simulink model "Optimized_wind_farm_with_dynamic_grid"  (R2015b)
settings: Solver=FixedStepAuto  StartTime=0.0  StopTime=24  FixedStep=Ts  RelTol=1e-3
undefined symbols (not defined in the file): Ts
libraries: powerlib x52, simulink x38, powerlib_meascontrol x30, powerlib_extras x4, sps_avr x1
(part 1 of 3)
settings Model: SimulationMode=accelerator  Creator=Eren  LastModifiedBy=Eren

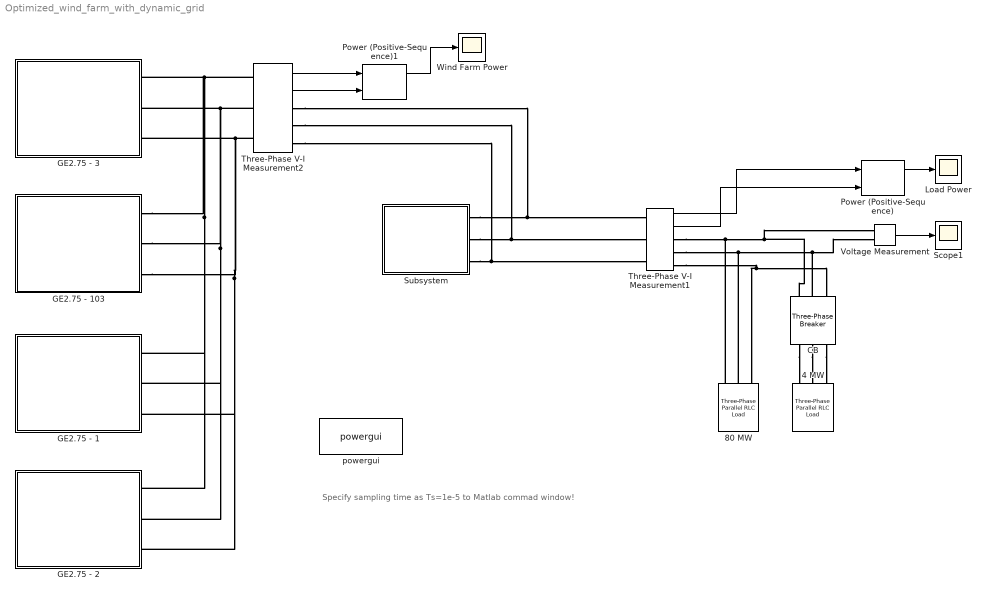
== system Optimized_wind_farm_with_dynamic_grid ==
  note: Specify sampling time as Ts=1e-5 to Matlab commad window!
  4 MW : powerlib/Elements/Three-Phase Parallel RLC Load  LConnTagsString=A|B|C  Configuration=Y (grounded)  NominalVoltage=690  Vabc=[1e3 1e3 1e3]  Vabcp=[1e3 1e3 1e3]  NominalFrequency=50  UnbalancedPower=off  ActivePower=8e6  InductivePower=0  CapacitivePower=0  Pabc=[10e3 9e3 11e3]  QLabc=[100 90 110]  QCabc=[100 90 110]  Pabcp=[10e3 9e3 11e3]  QLabcp=[100 90 110]  QCabcp=[100 90 110]  Measurements=None  LoadType=constant PQ
  80 MW : powerlib/Elements/Three-Phase Parallel RLC Load  LConnTagsString=A|B|C  Configuration=Y (grounded)  NominalVoltage=690  Vabc=[1e3 1e3 1e3]  Vabcp=[1e3 1e3 1e3]  NominalFrequency=50  UnbalancedPower=off  ActivePower=80e6  InductivePower=0  CapacitivePower=0  Pabc=[10e3 9e3 11e3]  QLabc=[100 90 110]  QCabc=[100 90 110]  Pabcp=[10e3 9e3 11e3]  QLabcp=[100 90 110]  QCabcp=[100 90 110]  Measurements=None  LoadType=constant PQ
  CB : powerlib/Elements/Three-Phase Breaker  InitialState=open  SwitchA=on  SwitchB=on  SwitchC=on  SwitchTimes=10  External=off  BreakerResistance=0.01  SnubberResistance=1e6  SnubberCapacitance=inf  Measurements=None
  GE2.75 - 1 : Subsystem  mask{Prated=2.75e6, R=51.5, windspeed=9, Jtotal=1058.2, p=1.225, startuptime=5, winit=-160, gear=117.4, wmax=2*pi*(1735/60), fluxlinkage=4, pgen=2, Ld=10e-4, Lq=10.5e-4, Rs=1e-10, drivefreq=10e3, fnom=50, Srated=3.04e6, Vdcset=2500, Cdc=27e-3, Lfilter=2e-4}
      mask prompts: Prated "Turbine Power (W)"; R "Blade Radius"; windspeed "Wind Speed"; Jtotal "Total Inertia"; p "Air Density"; startuptime "Turbine Start-up Time"; winit "Initial Generator Speed"; gear "Gearbox Ratio"; wmax "Max Generator Speed"; fluxlinkage "Flux Linkage"; pgen "Generator Pole Pairs"; Ld "Ld (H)"; Lq "Lq(H)"; Rs "Stator Resistance"; drivefreq "Drive Frequency"; fnom "Nominal Grid Frequency"; Srated "Drive Apparent Power"; Vdcset "DC Link Voltage"; Cdc "DC Link Capacitance"; Lfilter "Lfilter (H)"
      mask Display: image(imread('gepic.jpg'))
  GE2.75 - 103 : Subsystem  mask{Prated=2.75e6, R=51.5, windspeed=9, Jtotal=1058.2, p=1.225, startuptime=5, winit=-160, gear=117.4, wmax=2*pi*(1735/60), fluxlinkage=4, pgen=2, Ld=10e-4, Lq=10.5e-4, Rs=1e-10, drivefreq=10e3, fnom=50, Srated=3.04e6, Vdcset=2500, Cdc=27e-3, Lfilter=2e-4}
      mask prompts: Prated "Turbine Power (W)"; R "Blade Radius"; windspeed "Wind Speed"; Jtotal "Total Inertia"; p "Air Density"; startuptime "Turbine Start-up Time"; winit "Initial Generator Speed"; gear "Gearbox Ratio"; wmax "Max Generator Speed"; fluxlinkage "Flux Linkage"; pgen "Generator Pole Pairs"; Ld "Ld (H)"; Lq "Lq(H)"; Rs "Stator Resistance"; drivefreq "Drive Frequency"; fnom "Nominal Grid Frequency"; Srated "Drive Apparent Power"; Vdcset "DC Link Voltage"; Cdc "DC Link Capacitance"; Lfilter "Lfilter (H)"
      mask Display: image(imread('gepic.jpg'))
  GE2.75 - 2 : Subsystem  mask{Prated=2.75e6, R=51.5, windspeed=9, Jtotal=1058.2, p=1.225, startuptime=5, winit=-160, gear=117.4, wmax=2*pi*(1735/60), fluxlinkage=4, pgen=2, Ld=10e-4, Lq=10.5e-4, Rs=1e-10, drivefreq=10e3, fnom=50, Srated=3.04e6, Vdcset=2500, Cdc=27e-3, Lfilter=2e-4}
      mask prompts: Prated "Turbine Power (W)"; R "Blade Radius"; windspeed "Wind Speed"; Jtotal "Total Inertia"; p "Air Density"; startuptime "Turbine Start-up Time"; winit "Initial Generator Speed"; gear "Gearbox Ratio"; wmax "Max Generator Speed"; fluxlinkage "Flux Linkage"; pgen "Generator Pole Pairs"; Ld "Ld (H)"; Lq "Lq(H)"; Rs "Stator Resistance"; drivefreq "Drive Frequency"; fnom "Nominal Grid Frequency"; Srated "Drive Apparent Power"; Vdcset "DC Link Voltage"; Cdc "DC Link Capacitance"; Lfilter "Lfilter (H)"
      mask Display: image(imread('gepic.jpg'))
  GE2.75 - 3 : Subsystem  mask{Prated=2.75e6, R=51.5, windspeed=9, Jtotal=1058.2, p=1.225, startuptime=5, winit=-160, gear=117.4, wmax=2*pi*(1735/60), fluxlinkage=4, pgen=2, Ld=10e-4, Lq=10.5e-4, Rs=1e-10, drivefreq=10e3, fnom=50, Srated=3.04e6, Vdcset=2500, Cdc=27e-3, Lfilter=2e-4}
      mask prompts: Prated "Turbine Power (W)"; R "Blade Radius"; windspeed "Wind Speed"; Jtotal "Total Inertia"; p "Air Density"; startuptime "Turbine Start-up Time"; winit "Initial Generator Speed"; gear "Gearbox Ratio"; wmax "Max Generator Speed"; fluxlinkage "Flux Linkage"; pgen "Generator Pole Pairs"; Ld "Ld (H)"; Lq "Lq(H)"; Rs "Stator Resistance"; drivefreq "Drive Frequency"; fnom "Nominal Grid Frequency"; Srated "Drive Apparent Power"; Vdcset "DC Link Voltage"; Cdc "DC Link Capacitance"; Lfilter "Lfilter (H)"
      mask Display: image(imread('gepic.jpg'))
  Load Power : Scope
  Power (Positive-Sequence) : powerlib_meascontrol/Measurements/Power (Positive-Sequence)  Freq=50  Vinit=[0, 0]  Iinit=[0, 0]  Ts=0
  Power (Positive-Sequence)1 : powerlib_meascontrol/Measurements/Power (Positive-Sequence)  Freq=50  Vinit=[0, 0]  Iinit=[0, 0]  Ts=0
  Scope1 : Scope
  Subsystem : Subsystem
  Three-Phase V-I Measurement1 : powerlib/Measurements/Three-Phase V-I Measurement  VoltageMeasurement=phase-to-ground  SetLabelV=off  LabelV=Vsabc  Vpu=off  VpuLL=on  CurrentMeasurement=yes  SetLabelI=off  LabelI=Isabc  Ipu=off  Pbase=100e6  Vbase=690  OutputType=Complex  PhasorSimulation=off  PSBequivalent=0
  Three-Phase V-I Measurement2 : powerlib/Measurements/Three-Phase V-I Measurement  VoltageMeasurement=phase-to-ground  SetLabelV=off  LabelV=Vsabc  Vpu=off  VpuLL=on  CurrentMeasurement=yes  SetLabelI=off  LabelI=Isabc  Ipu=off  Pbase=100e6  Vbase=690  OutputType=Complex  PhasorSimulation=off  PSBequivalent=0
  Voltage Measurement : powerlib/Measurements/Voltage Measurement  PhasorSimulation=off  OutputType=Complex  PSBequivalent=0
  Wind Farm Power : Scope
  powergui : powerlib/powergui  Priority=2  SimulationMode=Discrete  SolverType=Tustin  SampleTime=Ts  frequency=60  SPID=off  DisableSnubberDevices=off  DisableRonSwitches=off  DisableVfSwitches=off  SwTol=0  DisplayEquations=off  Interpol=off  ExternalGateDelay=off  methode=off  Ts=0  FunctionMessages=off  echomessages=off  HookPort=off  EnableUseOfTLC=off  x0status=blocks  frequencyindice=50  Pbase=100e6  ErrMax=1e-4  Iterations=50  UnitsV=kV  UnitsW=MW  buscounter=0  RestoreLinks=warning  ResistiveCurrentMeasurement=off  Frange=[0:2:500]  Ylog=off  Xlog=on  ShowGrid=off  save=off  variable=ZData  structure=0  ZoomFFT=on  StartTime=0.0  cycles=1  DisplayStyle=1  fundamental=60  FreqAxis=off  MaxFrequency=1000  frequencyindicesteady=1  RmsSteady=1  display=off
  wires:
  Voltage Measurement/1 -> Scope1/1
  Three-Phase V-I Measurement1/1 -> Power (Positive-Sequence)/1
  Three-Phase V-I Measurement1/2 -> Power (Positive-Sequence)/2
  Power (Positive-Sequence)/1 -> Load Power/1
  Power (Positive-Sequence)1/1 -> Wind Farm Power/1
  Three-Phase V-I Measurement2/1 -> Power (Positive-Sequence)1/1
  Three-Phase V-I Measurement2/2 -> Power (Positive-Sequence)1/2
  connections:
  80 MW/LConn1 -- CB/RConn1 -- Voltage Measurement/LConn1 -- Three-Phase V-I Measurement1/RConn1
  80 MW/LConn2 -- CB/RConn2 -- Voltage Measurement/LConn2 -- Three-Phase V-I Measurement1/RConn2
  Three-Phase V-I Measurement1/RConn3 -- CB/RConn3 -- 80 MW/LConn3
  CB/LConn2 -- 4 MW/LConn2
  CB/LConn1 -- 4 MW/LConn1
  CB/LConn3 -- 4 MW/LConn3
  Subsystem/RConn3 -- Three-Phase V-I Measurement2/RConn3 -- Three-Phase V-I Measurement1/LConn3
  Subsystem/RConn1 -- Three-Phase V-I Measurement2/RConn1 -- Three-Phase V-I Measurement1/LConn1
  Subsystem/RConn2 -- Three-Phase V-I Measurement1/LConn2 -- Three-Phase V-I Measurement2/RConn2
  Three-Phase V-I Measurement2/LConn1 -- GE2.75 - 103/RConn1 -- GE2.75 - 2/RConn1 -- GE2.75 - 1/RConn1 -- GE2.75 - 3/RConn1
  Three-Phase V-I Measurement2/LConn2 -- GE2.75 - 103/RConn2 -- GE2.75 - 2/RConn2 -- GE2.75 - 1/RConn2 -- GE2.75 - 3/RConn2
  Three-Phase V-I Measurement2/LConn3 -- GE2.75 - 103/RConn3 -- GE2.75 - 2/RConn3 -- GE2.75 - 1/RConn3 -- GE2.75 - 3/RConn3

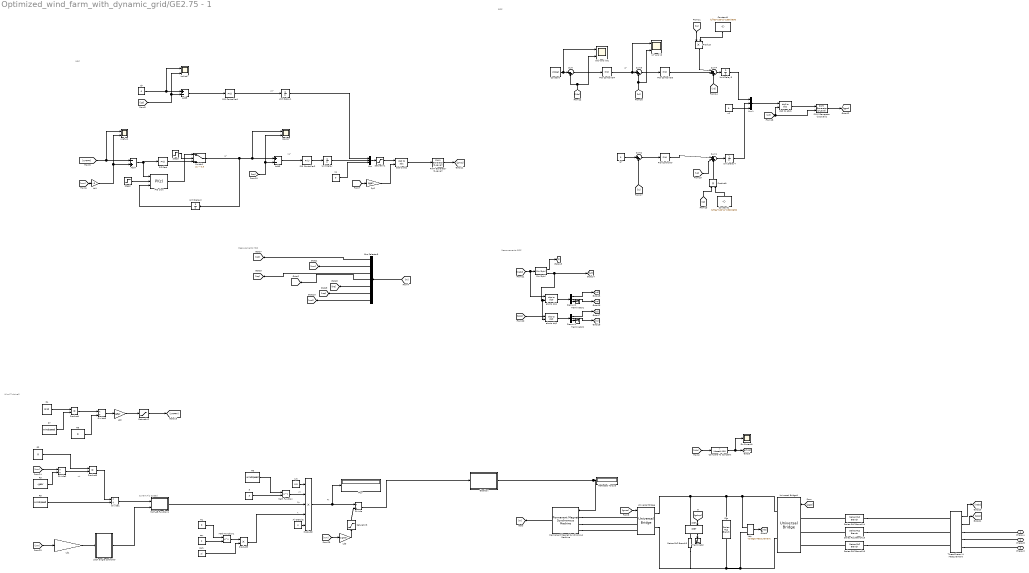
== system Optimized_wind_farm_with_dynamic_grid/GE2.75 - 1 ==
  note: Wind Turbine2
  note: Measurements GSC
  note: GSC
  note: MSC
  note: Measurements MSC
  note: Vd*
  note: Vq*
  note: iq*
  note: id*
  note: Current Tip Speed
  note: wt
  note: A
  note: Cp
  note: v3
  note: Pt
  1/2 : Constant  Value=0.5
  3 : Constant  Value=3
  Add3 : Sum  Inputs=+-
  Add5 : Sum  Inputs=+-
  Add7 : Sum  Inputs=-+
  Air Density : Constant  Value=p
  Bus Selector5 : BusSelector  OutputSignals=Stator current is_d (A),Rotor speed wm (rad/s),Stator current is_q (A),Rotor angle thetam (rad),Electromagnetic torque Te (N*m),Stator voltage Vs_q (V),Stator voltage Vs_d (V)
  Cdc : powerlib/Elements/Series RLC Branch  LConnTagsString=__new0  RConnTagsString=__new0  BranchType=C  Resistance=1  Inductance=1e-4  SetiL0=off  InitialCurrent=0  Capacitance=Cdc  Setx0=off  InitialVoltage=0  Measurements=None
  Compare To Constant : simulink/Logic and Bit Operations/Compare To Constant  relop=>  const=Vdcset+100  OutDataTypeStr=boolean
  Constant : Constant  Value=Vdcset
  Constant1 : Constant  Value=(Lfilter*100*pi*2300)/690
  Constant2 : Constant  Value=(Lfilter*100*pi*2300)/690
  Dc Current1 : Scope
  Demux1 : Demux  Outputs=3
  Demux2 : Demux  Outputs=3
  Divide{,1..3} (4 alike) : Product  Inputs=*/
  Gearbox : Subsystem
  IGBT : powerlib/Power Electronics/IGBT  Ron=0.001  Lon=0  Vf=1  Tf=1e-6  Tt=2e-6  IC=0  Rs=1e5  Cs=inf  Measurements=on
  Id* : Constant  Value=0
  Ld1 : Gain  Gain=-pgen/(2*fnom*pi)
  Ld2 : Gain  Gain=gear
  Ld3 : Gain  Gain=-1/gear
  Ld4 : Gain  Gain=-1
  MATLAB Function1 : MATLAB Function  TreatAsAtomicUnit=on
  Math Function : Math  Operator=pow  SaturateOnIntegerOverflow=on
  Math Function1 : Math  Operator=pow  SaturateOnIntegerOverflow=on
  Mux : Mux  Inputs=3
  Mux1 : Mux  Inputs=3
  PID Controller : simulink/Continuous/PID Controller  Controller=PI  TimeDomain=Continuous-time  SampleTime=-1  IntegratorMethod=Forward Euler  FilterMethod=Forward Euler  Form=Parallel  UseFilter=on  ControllerParametersSource=internal  P=15  I=1  D=0  N=100  InitialConditionSource=internal  InitialConditionForIntegrator=0  InitialConditionForFilter=0  ExternalReset=none  LimitOutput=on  UpperSaturationLimit=2  LowerSaturationLimit=-2  LinearizeAsGain=on  AntiWindupMode=none  Kb=1  TrackingMode=off  Kt=1  PParamMin=[]  PParamMax=[]  IParamMin=[]  IParamMax=[]  DParamMin=[]  DParamMax=[]  NParamMin=[]  NParamMax=[]  KbParamMin=[]  KbParamMax=[]  KtParamMin=[]  KtParamMax=[]  POutMin=[]  POutMax=[]  IOutMin=[]  IOutMax=[]  DOutMin=[]  DOutMax=[]  NOutMin=[]  NOutMax=[]  KbOutMin=[]  KbOutMax=[]  KtOutMin=[]  KtOutMax=[]  IntegratorOutMin=[]  IntegratorOutMax=[]  FilterOutMin=[]  FilterOutMax=[]  SumOutMin=[]  SumOutMax=[]  SumI1OutMin=[]  SumI1OutMax=[]  SumI2OutMin=[]  SumI2OutMax=[]  SumI3OutMin=[]  SumI3OutMax=[]  SumDOutMin=[]  SumDOutMax=[]  SaturationOutMin=[]  SaturationOutMax=[]  IntegratorContinuousStateAttributes=''  IntegratorStateMustResolveToSignalObject=off  IntegratorRTWStateStorageClass=Auto  FilterContinuousStateAttributes=''  FilterStateMustResolveToSignalObject=off  FilterRTWStateStorageClass=Auto  DifferentiatorICPrevScaledInput=0  DifferentiatorOutMin=[]  DifferentiatorOutMax=[]
  PID Controller1 : simulink/Continuous/PID Controller  Controller=PI  TimeDomain=Discrete-time  SampleTime=-1  IntegratorMethod=Forward Euler  FilterMethod=Forward Euler  Form=Parallel  UseFilter=on  ControllerParametersSource=internal  P=0.25  I=0.05  D=0  N=100  InitialConditionSource=internal  InitialConditionForIntegrator=0  InitialConditionForFilter=0  ExternalReset=none  LimitOutput=off  UpperSaturationLimit=inf  LowerSaturationLimit=-inf  LinearizeAsGain=on  AntiWindupMode=none  Kb=1  TrackingMode=off  Kt=1  PParamMin=[]  PParamMax=[]  IParamMin=[]  IParamMax=[]  DParamMin=[]  DParamMax=[]  NParamMin=[]  NParamMax=[]  KbParamMin=[]  KbParamMax=[]  KtParamMin=[]  KtParamMax=[]  POutMin=[]  POutMax=[]  IOutMin=[]  IOutMax=[]  DOutMin=[]  DOutMax=[]  NOutMin=[]  NOutMax=[]  KbOutMin=[]  KbOutMax=[]  KtOutMin=[]  KtOutMax=[]  IntegratorOutMin=[]  IntegratorOutMax=[]  FilterOutMin=[]  FilterOutMax=[]  SumOutMin=[]  SumOutMax=[]  SumI1OutMin=[]  SumI1OutMax=[]  SumI2OutMin=[]  SumI2OutMax=[]  SumI3OutMin=[]  SumI3OutMax=[]  SumDOutMin=[]  SumDOutMax=[]  SaturationOutMin=[]  SaturationOutMax=[]  IntegratorContinuousStateAttributes=''  IntegratorStateMustResolveToSignalObject=off  IntegratorRTWStateStorageClass=Auto  FilterContinuousStateAttributes=''  FilterStateMustResolveToSignalObject=off  FilterRTWStateStorageClass=Auto  DifferentiatorICPrevScaledInput=0  DifferentiatorOutMin=[]  DifferentiatorOutMax=[]
  PID Controller2 : simulink/Continuous/PID Controller  Controller=PI  TimeDomain=Discrete-time  SampleTime=-1  IntegratorMethod=Forward Euler  FilterMethod=Forward Euler  Form=Parallel  UseFilter=on  ControllerParametersSource=internal  P=1  I=0.05  D=0  N=100  InitialConditionSource=internal  InitialConditionForIntegrator=0  InitialConditionForFilter=0  ExternalReset=none  LimitOutput=off  UpperSaturationLimit=inf  LowerSaturationLimit=-inf  LinearizeAsGain=on  AntiWindupMode=none  Kb=1  TrackingMode=off  Kt=1  PParamMin=[]  PParamMax=[]  IParamMin=[]  IParamMax=[]  DParamMin=[]  DParamMax=[]  NParamMin=[]  NParamMax=[]  KbParamMin=[]  KbParamMax=[]  KtParamMin=[]  KtParamMax=[]  POutMin=[]  POutMax=[]  IOutMin=[]  IOutMax=[]  DOutMin=[]  DOutMax=[]  NOutMin=[]  NOutMax=[]  KbOutMin=[]  KbOutMax=[]  KtOutMin=[]  KtOutMax=[]  IntegratorOutMin=[]  IntegratorOutMax=[]  FilterOutMin=[]  FilterOutMax=[]  SumOutMin=[]  SumOutMax=[]  SumI1OutMin=[]  SumI1OutMax=[]  SumI2OutMin=[]  SumI2OutMax=[]  SumI3OutMin=[]  SumI3OutMax=[]  SumDOutMin=[]  SumDOutMax=[]  SaturationOutMin=[]  SaturationOutMax=[]  IntegratorContinuousStateAttributes=''  IntegratorStateMustResolveToSignalObject=off  IntegratorRTWStateStorageClass=Auto  FilterContinuousStateAttributes=''  FilterStateMustResolveToSignalObject=off  FilterRTWStateStorageClass=Auto  DifferentiatorICPrevScaledInput=0  DifferentiatorOutMin=[]  DifferentiatorOutMax=[]
  PID Controller3 : simulink/Continuous/PID Controller  Controller=PI  TimeDomain=Continuous-time  SampleTime=-1  IntegratorMethod=Forward Euler  FilterMethod=Forward Euler  Form=Parallel  UseFilter=on  ControllerParametersSource=internal  P=100  I=5  D=0  N=100  InitialConditionSource=internal  InitialConditionForIntegrator=0  InitialConditionForFilter=0  ExternalReset=none  LimitOutput=on  UpperSaturationLimit=1.5  LowerSaturationLimit=-1.5  LinearizeAsGain=on  AntiWindupMode=none  Kb=1  TrackingMode=off  Kt=1  PParamMin=[]  PParamMax=[]  IParamMin=[]  IParamMax=[]  DParamMin=[]  DParamMax=[]  NParamMin=[]  NParamMax=[]  KbParamMin=[]  KbParamMax=[]  KtParamMin=[]  KtParamMax=[]  POutMin=[]  POutMax=[]  IOutMin=[]  IOutMax=[]  DOutMin=[]  DOutMax=[]  NOutMin=[]  NOutMax=[]  KbOutMin=[]  KbOutMax=[]  KtOutMin=[]  KtOutMax=[]  IntegratorOutMin=[]  IntegratorOutMax=[]  FilterOutMin=[]  FilterOutMax=[]  SumOutMin=[]  SumOutMax=[]  SumI1OutMin=[]  SumI1OutMax=[]  SumI2OutMin=[]  SumI2OutMax=[]  SumI3OutMin=[]  SumI3OutMax=[]  SumDOutMin=[]  SumDOutMax=[]  SaturationOutMin=[]  SaturationOutMax=[]  IntegratorContinuousStateAttributes=''  IntegratorStateMustResolveToSignalObject=off  IntegratorRTWStateStorageClass=Auto  FilterContinuousStateAttributes=''  FilterStateMustResolveToSignalObject=off  FilterRTWStateStorageClass=Auto  DifferentiatorICPrevScaledInput=0  DifferentiatorOutMin=[]  DifferentiatorOutMax=[]
  PID Controller4 : simulink/Continuous/PID Controller  Controller=PI  TimeDomain=Continuous-time  SampleTime=-1  IntegratorMethod=Forward Euler  FilterMethod=Forward Euler  Form=Parallel  UseFilter=on  ControllerParametersSource=internal  P=0.004  I=0.04  D=0  N=100  InitialConditionSource=internal  InitialConditionForIntegrator=0  InitialConditionForFilter=0  ExternalReset=none  LimitOutput=on  UpperSaturationLimit=1.2  LowerSaturationLimit=1e-6  LinearizeAsGain=on  AntiWindupMode=none  Kb=1  TrackingMode=off  Kt=1  PParamMin=[]  PParamMax=[]  IParamMin=[]  IParamMax=[]  DParamMin=[]  DParamMax=[]  NParamMin=[]  NParamMax=[]  KbParamMin=[]  KbParamMax=[]  KtParamMin=[]  KtParamMax=[]  POutMin=[]  POutMax=[]  IOutMin=[]  IOutMax=[]  DOutMin=[]  DOutMax=[]  NOutMin=[]  NOutMax=[]  KbOutMin=[]  KbOutMax=[]  KtOutMin=[]  KtOutMax=[]  IntegratorOutMin=[]  IntegratorOutMax=[]  FilterOutMin=[]  FilterOutMax=[]  SumOutMin=[]  SumOutMax=[]  SumI1OutMin=[]  SumI1OutMax=[]  SumI2OutMin=[]  SumI2OutMax=[]  SumI3OutMin=[]  SumI3OutMax=[]  SumDOutMin=[]  SumDOutMax=[]  SaturationOutMin=[]  SaturationOutMax=[]  IntegratorContinuousStateAttributes=''  IntegratorStateMustResolveToSignalObject=off  IntegratorRTWStateStorageClass=Auto  FilterContinuousStateAttributes=''  FilterStateMustResolveToSignalObject=off  FilterRTWStateStorageClass=Auto  DifferentiatorICPrevScaledInput=0  DifferentiatorOutMin=[]  DifferentiatorOutMax=[]
  PID fast : simulink/Continuous/PID Controller  Controller=PI  TimeDomain=Discrete-time  SampleTime=-1  IntegratorMethod=Forward Euler  FilterMethod=Forward Euler  Form=Parallel  UseFilter=on  ControllerParametersSource=internal  P=750  I=1000  D=0  N=100  InitialConditionSource=internal  InitialConditionForIntegrator=0  InitialConditionForFilter=0  ExternalReset=none  LimitOutput=on  UpperSaturationLimit=1255  LowerSaturationLimit=200  LinearizeAsGain=on  AntiWindupMode=none  Kb=1  TrackingMode=off  Kt=1  PParamMin=[]  PParamMax=[]  IParamMin=[]  IParamMax=[]  DParamMin=[]  DParamMax=[]  NParamMin=[]  NParamMax=[]  KbParamMin=[]  KbParamMax=[]  KtParamMin=[]  KtParamMax=[]  POutMin=[]  POutMax=[]  IOutMin=[]  IOutMax=[]  DOutMin=[]  DOutMax=[]  NOutMin=[]  NOutMax=[]  KbOutMin=[]  KbOutMax=[]  KtOutMin=[]  KtOutMax=[]  IntegratorOutMin=[]  IntegratorOutMax=[]  FilterOutMin=[]  FilterOutMax=[]  SumOutMin=[]  SumOutMax=[]  SumI1OutMin=[]  SumI1OutMax=[]  SumI2OutMin=[]  SumI2OutMax=[]  SumI3OutMin=[]  SumI3OutMax=[]  SumDOutMin=[]  SumDOutMax=[]  SaturationOutMin=[]  SaturationOutMax=[]  IntegratorContinuousStateAttributes=''  IntegratorStateMustResolveToSignalObject=off  IntegratorRTWStateStorageClass=Auto  FilterContinuousStateAttributes=''  FilterStateMustResolveToSignalObject=off  FilterRTWStateStorageClass=Auto  DifferentiatorICPrevScaledInput=0  DifferentiatorOutMin=[]  DifferentiatorOutMax=[]
  PID slow : simulink/Continuous/PID Controller  Controller=PI  TimeDomain=Discrete-time  SampleTime=-1  IntegratorMethod=Forward Euler  FilterMethod=Forward Euler  Form=Parallel  UseFilter=on  ControllerParametersSource=internal  P=30  I=1.6  D=0  N=100  InitialConditionSource=external  InitialConditionForIntegrator=0  InitialConditionForFilter=0  ExternalReset=rising  LimitOutput=on  UpperSaturationLimit=1255  LowerSaturationLimit=200  LinearizeAsGain=on  AntiWindupMode=none  Kb=1  TrackingMode=off  Kt=1  PParamMin=[]  PParamMax=[]  IParamMin=[]  IParamMax=[]  DParamMin=[]  DParamMax=[]  NParamMin=[]  NParamMax=[]  KbParamMin=[]  KbParamMax=[]  KtParamMin=[]  KtParamMax=[]  POutMin=[]  POutMax=[]  IOutMin=[]  IOutMax=[]  DOutMin=[]  DOutMax=[]  NOutMin=[]  NOutMax=[]  KbOutMin=[]  KbOutMax=[]  KtOutMin=[]  KtOutMax=[]  IntegratorOutMin=[]  IntegratorOutMax=[]  FilterOutMin=[]  FilterOutMax=[]  SumOutMin=[]  SumOutMax=[]  SumI1OutMin=[]  SumI1OutMax=[]  SumI2OutMin=[]  SumI2OutMax=[]  SumI3OutMin=[]  SumI3OutMax=[]  SumDOutMin=[]  SumDOutMax=[]  SaturationOutMin=[]  SaturationOutMax=[]  IntegratorContinuousStateAttributes=''  IntegratorStateMustResolveToSignalObject=off  IntegratorRTWStateStorageClass=Auto  FilterContinuousStateAttributes=''  FilterStateMustResolveToSignalObject=off  FilterRTWStateStorageClass=Auto  DifferentiatorICPrevScaledInput=0  DifferentiatorOutMin=[]  DifferentiatorOutMax=[]
  PLL (3ph) : powerlib_meascontrol/PLL/PLL (3ph)  Fmin=45  Par_Init=[0, 50]  ParK=[180, 3200, 1]  TcD=1e-4  MaxRateChangeFreq=12  FilterCutOffFreq=25  Ts=Ts  AGC=on
  PWM Generator (2-Level) : powerlib_meascontrol/Pulse & Signal Generators/PWM Generator (2-Level)  ModulatorType=Three-phase bridge (6 pulses)  ModulatorMode=Unsynchronized  Fc=drivefreq  Pc=90  nF=60  MinMax="[ -1  1 ]"  SamplingTechnique=Natural  ModulatingSignals=off  m=0.8  Freq=60  Phase=0  Ts=Ts  ShowCarrierOutport=off
  PWM Generator (2-Level)2 : powerlib_meascontrol/Pulse & Signal Generators/PWM Generator (2-Level)  ModulatorType=Three-phase bridge (6 pulses)  ModulatorMode=Synchronized  Fc=50*60  Pc=90  nF=500  MinMax="[ -1  1 ]"  SamplingTechnique=Natural  ModulatingSignals=off  m=0.8  Freq=60  Phase=0  Ts=Ts  ShowCarrierOutport=off
  Permanent Magnet Synchronous Machine : powerlib/Machines/Permanent Magnet Synchronous Machine  NbPhases=3  FluxDistribution=Sinusoidal  RotorType=Salient-pole  MechanicalLoad=Torque Tm  PresetModel=No  ShowDetailedParameters=on  MeasurementBus=off  Resistance=Rs  Inductance=8.5e-3  dqInductances=[Ld,Lq]  La=Lq  MachineConstant=Flux linkage established by magnets (V.s)  Flux=fluxlinkage  VoltageCst=1451.0395  TorqueCst=12  Flat=120  Mechanical=[Jtotal 1.349e-05 pgen 0]  PolePairs=2  InitialConditions=[winit,0, 0,0]  InitialConditions5ph=[0 0 0 0 0 0]  TsPowergui=0  TsBlock=-1  RefAngle=Aligned with phase A axis (original Park)
  Pp2 : Gain  Gain=pgen
  Product{,1,3..5} (5 alike) : Product
  Product2 : Product  Inputs=5
  Ptur : Display
  R1 : Constant  Value=R
  R2 : Constant  Value=R
  R3 : Constant  Value=-gear
  R4 : Constant  Value=8.12
  R5 : Constant  Value=windspeed
  R6 : Constant  Value=windspeed
  R7 : Constant  Value=windspeed
  R8 : Constant  Value=R
  Reflected Torque : Display
  Saturatin1 : Saturate  UpperLimit=2000  LowerLimit=-2000
  Saturatin2 : Saturate  UpperLimit=wmax  LowerLimit=1e-8
  Saturatin3 : Saturate  UpperLimit=inf  LowerLimit=1e-8
  Series RLC Branch14 : powerlib/Elements/Series RLC Branch  LConnTagsString=__new0  RConnTagsString=__new0  BranchType=L  Resistance=1  Inductance=Lfilter  SetiL0=off  InitialCurrent=0  Capacitance=1e-6  Setx0=off  InitialVoltage=0  Measurements=None
  Series RLC Branch15 : powerlib/Elements/Series RLC Branch  LConnTagsString=__new0  RConnTagsString=__new0  BranchType=L  Resistance=1  Inductance=Lfilter  SetiL0=off  InitialCurrent=0  Capacitance=1e-6  Setx0=off  InitialVoltage=0  Measurements=None
  Series RLC Branch16 : powerlib/Elements/Series RLC Branch  LConnTagsString=__new0  RConnTagsString=__new0  BranchType=L  Resistance=1  Inductance=Lfilter  SetiL0=off  InitialCurrent=0  Capacitance=1e-6  Setx0=off  InitialVoltage=0  Measurements=None
  Series RLC Branch3 : powerlib/Elements/Series RLC Branch  LConnTagsString=__new0  RConnTagsString=__new0  BranchType=R  Resistance=1  Inductance=1e-4  SetiL0=off  InitialCurrent=0  Capacitance=Cdc  Setx0=off  InitialVoltage=0  Measurements=None
  Step2 : Step  Time=startuptime
  Step3 : Step  Time=startuptime
  Sum : Sum  Inputs=|-+
  Sum1 : Sum  Inputs=|+++
  Sum2 : Sum  Inputs=|+-
  Sum3 : Sum  Inputs=|+-
  Sum4 : Sum  Inputs=|-++
  Switch1 : Switch  Criteria=u2 > Threshold  Threshold=0.5
  Terminator : Terminator
  Terminator1 : Terminator
  Terminator2 : Terminator
  Three-Phase V-I Measurement : powerlib/Measurements/Three-Phase V-I Measurement  VoltageMeasurement=phase-to-ground  SetLabelV=off  LabelV=Vabc  Vpu=on  VpuLL=off  CurrentMeasurement=yes  SetLabelI=off  LabelI=Iabc  Ipu=on  Pbase=2.75e6  Vbase=690  OutputType=Complex  PhasorSimulation=off  PSBequivalent=0
  Unit Delay{,1..4} (5 alike) : UnitDelay  SampleTime=Ts
  Universal Bridge : powerlib/Power Electronics/Universal Bridge  Arms=3  SnubberResistance=1e5  SnubberCapacitance=inf  Device=IGBT / Diodes  Ron=1e-3  Lon=0  ForwardVoltages="[  0  0  ]"  ForwardVoltage=0  GTOparameters=[ 10e-6 , 20e-6 ]  IGBTparameters=[ 1e-6 , 2e-6 ]  Measurements=None  Measurements_2=None  converterType=Rectifier
  Universal Bridge1 : powerlib/Power Electronics/Universal Bridge  Arms=3  SnubberResistance=1e5  SnubberCapacitance=inf  Device=IGBT / Diodes  Ron=0.00001  Lon=0  ForwardVoltages="[  0  0  ]"  ForwardVoltage=0  GTOparameters=[ 10e-6 , 20e-6 ]  IGBTparameters=[ 0 , 0 ]  Measurements=None  Measurements_2=None  converterType=Rectifier
  Vdc : powerlib/Measurements/Voltage Measurement  PhasorSimulation=off  OutputType=Complex  PSBequivalent=0
  Vdc* and Vdc : Scope  NumInputPorts=2
  Vo : Constant  Value=0
  abc to dq1 : powerlib_meascontrol/Transformations/abc to dq0  Alignment=90 degrees behind phase A axis
  abc to dq2 : powerlib_meascontrol/Transformations/abc to dq0  Alignment=90 degrees behind phase A axis
  dq0 to abc : powerlib_meascontrol/Transformations/dq0 to abc  Alignment=Aligned with phase A axis
  dq0 to abc1 : powerlib_meascontrol/Transformations/dq0 to abc  Alignment=90 degrees behind phase A axis
  "id* and id " : Scope  NumInputPorts=2
  iq* : Constant  Value=0
  isd-isd* : Scope  NumInputPorts=2
  isq-isq* : Scope  NumInputPorts=2
  pitch angle controller : Subsystem
  sqr : Constant  Value=2
  sqr1 : Constant  Value=pi
  v0 : Constant  Value=0
  wref-w1 : Scope  NumInputPorts=2
  Phase A : PMIOPort  Port=1  Side=Right
  Phase B : PMIOPort  Port=2  Side=Right
  Phase C : PMIOPort  Port=3  Side=Right
  wires:
  Gearbox/1(Tt') -> Permanent Magnet Synchronous Machine/1, Reflected Torque/1
  Divide/1 -> Gearbox/1(Tt)
  [ggsc] -> Universal Bridge1/1
  Vdc/1 -> [Vdc]
  [Vdc] -> Compare To Constant/1
  Compare To Constant/1 -> Dc Current1/1, [gchop]
  [gchop] -> IGBT/1
  IGBT/1 -> Terminator/1
  [gmsc] -> Universal Bridge/1
  Permanent Magnet Synchronous Machine/1 -> [m]
  [m] -> Bus Selector5/1
  Bus Selector5/7 -> [vsd]  "<Stator voltage Vs_d (V)>"
  Bus Selector5/3 -> [isq]  "<Stator current is_q (A)>"
  Bus Selector5/1 -> [isd]  "<Stator current is_d (A)>"
  Bus Selector5/4 -> [thetam]  "<Rotor angle thetam (rad)>"
  Bus Selector5/5 -> [Te]  "<Electromagnetic torque Te (N*m)>"
  Bus Selector5/2 -> [wm]  "<Rotor speed wm (rad/s)>"
  Bus Selector5/6 -> [vsq]  "<Stator voltage Vs_q (V)>"
  PWM Generator (2-Level)/1 -> [gmsc]
  dq0 to abc/1 -> PWM Generator (2-Level)/1
  Unit Delay2/1 -> PID slow/3
  Switch1/1 -> Unit Delay2/1, isq-isq*/1, Add3/1
  Step3/1 -> Switch1/2
  PID slow/1 -> Switch1/1
  Step2/1 -> PID slow/2
  Ld4/1 -> Add7/2, wref-w1/2
  [wm] -> Ld4/1
  Unit Delay1/1 -> Mux/1
  Unit Delay/1 -> Mux/2
  PID fast/1 -> Switch1/3
  [isq] -> isq-isq*/2, Add3/2
  [isd] -> isd-isd*/2, Add5/2
  Id*/1 -> Add5/1, isd-isd*/1
  [wMPPT] -> wref-w1/1, Add7/1
  Add7/1 -> PID fast/1, PID slow/1
  PID Controller2/1 -> Unit Delay/1
  Saturatin1/1 -> dq0 to abc/1
  Pp2/1 -> dq0 to abc/2
  [thetam] -> Pp2/1
  PID Controller1/1 -> Unit Delay1/1
  Add5/1 -> PID Controller1/1
  Add3/1 -> PID Controller2/1
  Vo/1 -> Mux/3
  Mux/1 -> Saturatin1/1
  Product1/1 -> Sum1/3
  Product/1 -> Sum4/1
  [id] -> "id* and id "/2, Sum3/2
  [iq] -> Sum2/2
  Constant2/1 -> Product1/2
  [id] -> Product1/1
  Constant1/1 -> Product/2
  [iq] -> Product/1
  [vd] -> Sum4/3
  Unit Delay4/1 -> Mux1/2
  Unit Delay3/1 -> Mux1/1
  Constant/1 -> Vdc* and Vdc/1, Sum/1
  dq0 to abc1/1 -> PWM Generator (2-Level)2/1
  Sum/1 -> PID Controller4/1
  [Vdc] -> Vdc* and Vdc/2, Sum/2
  v0/1 -> Mux1/3
  Sum1/1 -> Unit Delay4/1
  [wt] -> dq0 to abc1/2, PWM Generator (2-Level)2/2
  Mux1/1 -> dq0 to abc1/1
  Sum4/1 -> Unit Delay3/1
  PID Controller3/1 -> Sum4/2
  Sum2/1 -> PID Controller/1
  [vq] -> Sum1/2
  PID Controller/1 -> Sum1/1
  PID Controller4/1 -> "id* and id "/1, Sum3/1
  Sum3/1 -> PID Controller3/1
  iq*/1 -> Sum2/1
  PWM Generator (2-Level)2/1 -> [ggsc]
  PLL (3ph)/1 -> [f]
  abc to dq2/1 -> Demux1/1
  abc to dq1/1 -> Demux2/1
  Demux1/2 -> [iq]
  Demux1/1 -> [id]
  Demux2/2 -> [vq]
  Demux2/1 -> [vd]
  [Iabc] -> abc to dq2/1
  PLL (3ph)/2 -> abc to dq2/2, abc to dq1/2, [wt]
  [Vabc] -> abc to dq1/1, PLL (3ph)/1
  Saturatin2/1 -> [wMPPT]
  Ld2/1 -> Saturatin2/1
  Divide3/1 -> Ld2/1
  R8/1 -> Divide3/2
  Product4/1 -> Divide3/1
  R7/1 -> Product4/2
  R4/1 -> Product4/1
  Saturatin3/1 -> Divide/2
  [wm] -> Ld1/1
  Ld1/1 -> pitch angle controller/1(wr)
  Product2/1 -> Ptur/1, Divide/1
  pitch angle controller/1(Beta) -> MATLAB Function1/2(B)
  R6/1 -> Math Function/1
  R3/1 -> Divide2/2
  MATLAB Function1/1(Cp) -> Product2/3
  Ld3/1 -> Saturatin3/1
  Divide2/1 -> Product5/2
  Divide1/1 -> MATLAB Function1/1(u)
  R5/1 -> Divide1/2
  Product5/1 -> Divide1/1
  [wm] -> Divide2/1
  R2/1 -> Product5/1
  3/1 -> Math Function/2
  R1/1 -> Math Function1/1
  sqr/1 -> Math Function1/2
  Math Function/1 -> Product2/2
  [wm] -> Ld3/1
  sqr1/1 -> Product3/2
  Math Function1/1 -> Product3/1
  Product3/1 -> Product2/4
  1/2/1 -> Product2/1
  Air Density/1 -> Product2/5
  Three-Phase V-I Measurement/1 -> [Vabc]
  Three-Phase V-I Measurement/2 -> [Iabc]
  Demux2/3 -> Terminator1/1
  Demux1/3 -> Terminator2/1
  connections:
  Three-Phase V-I Measurement/RConn1 -- Phase A/RConn1
  Three-Phase V-I Measurement/RConn2 -- Phase B/RConn1
  Three-Phase V-I Measurement/RConn3 -- Phase C/RConn1
  Permanent Magnet Synchronous Machine/LConn1 -- Universal Bridge/LConn1
  Permanent Magnet Synchronous Machine/LConn2 -- Universal Bridge/LConn2
  Series RLC Branch14/RConn1 -- Three-Phase V-I Measurement/LConn1
  Series RLC Branch16/RConn1 -- Three-Phase V-I Measurement/LConn3
  Series RLC Branch16/LConn1 -- Universal Bridge1/LConn3
  Series RLC Branch15/RConn1 -- Three-Phase V-I Measurement/LConn2
  Universal Bridge1/RConn2 -- Universal Bridge/RConn2 -- Series RLC Branch3/RConn1 -- Cdc/RConn1 -- Vdc/LConn2
  Permanent Magnet Synchronous Machine/LConn3 -- Universal Bridge/LConn3
  Series RLC Branch15/LConn1 -- Universal Bridge1/LConn2
  Series RLC Branch14/LConn1 -- Universal Bridge1/LConn1
  Universal Bridge/RConn1 -- IGBT/LConn1 -- Universal Bridge1/RConn1 -- Vdc/LConn1 -- Cdc/LConn1
  Series RLC Branch3/LConn1 -- IGBT/RConn1
